simulink model "ex11_2"  (Simulink 7.2)
settings: Solver=ode5  StartTime=0.0  StopTime=1  FixedStep=0.001  RelTol=1e-3
settings Model: Creator=Lenovo  LastModifiedBy=Lenovo

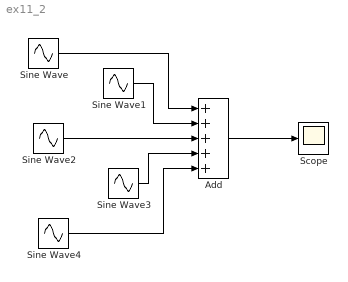
== system ex11_2 ==
  Add : Sum  Inputs=+++++  OutDataType=sfix(16)  OutScaling=2^-10
  Scope : Scope
  Sine Wave : Sin  Frequency=2*pi  SampleTime=0
  Sine Wave1 : Sin  Amplitude=1/3  Frequency=6*pi  SampleTime=0
  Sine Wave2 : Sin  Amplitude=1/5  Frequency=10*pi  SampleTime=0
  Sine Wave3 : Sin  Amplitude=1/7  Frequency=14*pi  SampleTime=0
  Sine Wave4 : Sin  Amplitude=1/9  Frequency=18*pi  SampleTime=0
  wires:
  Add/1 -> Scope/1
  Sine Wave2/1 -> Add/3
  Sine Wave3/1 -> Add/4
  Sine Wave4/1 -> Add/5
  Sine Wave1/1 -> Add/2
  Sine Wave/1 -> Add/1
